simulink model "simulink1"  (R2024a)
settings: Solver=VariableStepAuto  StartTime=0.0  StopTime=10.0  RelTol=1e-3
settings Model: Creator=parsaofrivia  LastModifiedBy=parsaofrivia

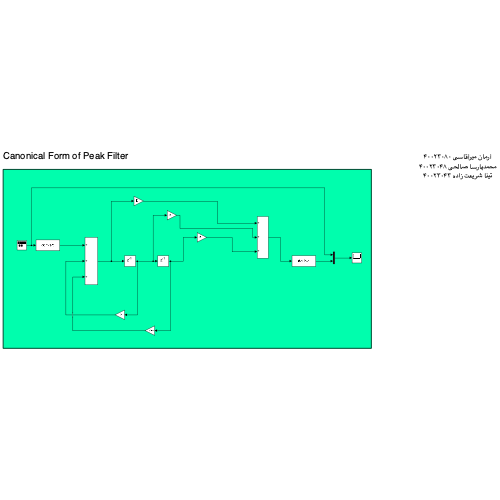
[thumbnail: Simulink's stored preview of the top-level diagram]
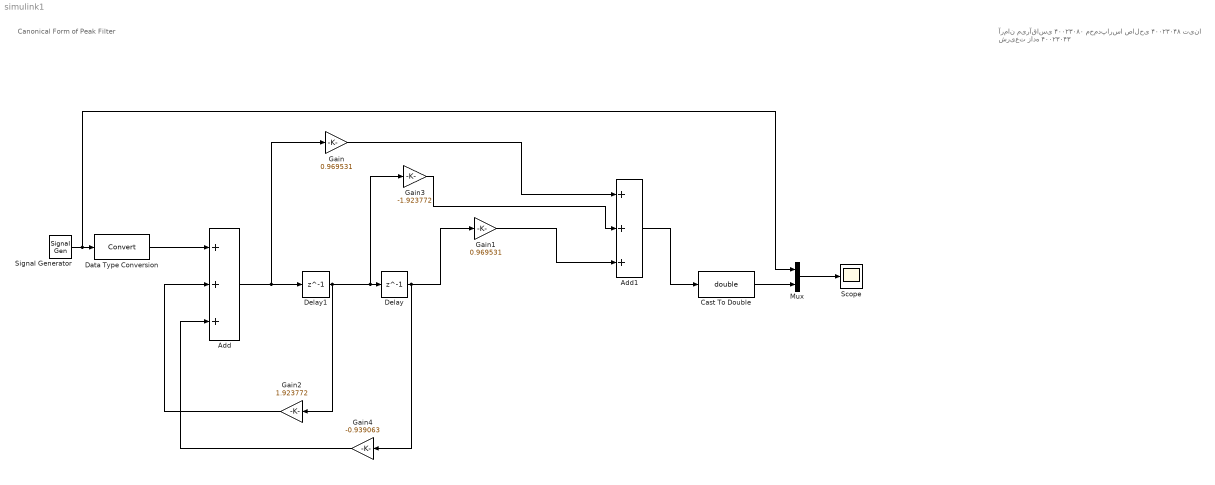
== system simulink1 ==
  note: آرمان میرآقاسی ۴۰۰۲۳۰۸۰
      | محمدپارسا صالحی ۴۰۰۲۳۰۴۸
      | تینا شریعت زاده ۴۰۰۲۳۰۴۳
  note: Canonical Form of Peak Filter
  Add : Sum  Inputs=+++
  Add1 : Sum  Inputs=+++
  Cast To Double : DataTypeConversion  OutDataTypeStr=double  SaturateOnIntegerOverflow=off  RndMeth=Floor
  Data Type Conversion : DataTypeConversion  SaturateOnIntegerOverflow=off  RndMeth=Floor
  Delay : Delay  DelayLength=1  InitialCondition=0
  Delay1 : Delay  DelayLength=1  InitialCondition=0
  Gain : Gain  Gain=0.969531
  Gain1 : Gain  Gain=0.969531
  Gain2 : Gain  Gain=1.923772
  Gain3 : Gain  Gain=-1.923772
  Gain4 : Gain  Gain=-0.939063
  Mux : Mux  Inputs=2
  Scope : Scope
  Signal Generator : SignalGenerator  Frequency=400  Units=rad/sec
  wires:
  Signal Generator/1 -> Mux/1, Data Type Conversion/1
  Data Type Conversion/1 -> Add/1
  Add/1 -> Delay1/1, Gain/1
  Delay1/1 -> Gain2/1, Gain3/1, Delay/1
  Delay/1 -> Gain4/1, Gain1/1
  Gain/1 -> Add1/1
  Gain3/1 -> Add1/2
  Gain1/1 -> Add1/3
  Add1/1 -> Cast To Double/1
  Gain2/1 -> Add/2
  Gain4/1 -> Add/3
  Cast To Double/1 -> Mux/2
  Mux/1 -> Scope/1
